simulink model "ADSBMonitor2020"  (R2020b)
settings: Solver=FixedStepDiscrete  StartTime=0.0  StopTime=inf  RelTol=1e-3
PreLoadFcn:
  | radioSampleRate = 2.4e6;
  | adsbParam = helperAdsbConfig(radioSampleRate);
  | load dataAdsbBusObjects
  | LaunchMap = 0;
  | LogData = 0;
  | BaudRate=9600;
InitFcn:
  | load dataAdsbBusObjects
  | helperAdsbCheckModelParams;
libraries: simrfV2util1 x3, simulink x2, instrumentlib x2, ADSBExampleLib x2, commsource2 x1, simrfV2systems x1, sdrrlib x1
CloseFcn:
  | hFig = findall(0, 'Type', 'figure', 'Tag', 'ADS-B Aircraft Tracking');
  | if ishghandle(hFig)
  | close(hFig);
  | end
  | clear hFig
settings Model: Creator=The MathWorks, Inc.  LastModifiedBy=Michael
settings DataIOCC: LimitDataPoints=on  SaveFormat=Array  SaveOutput=off  SaveTime=off  ReturnWorkspaceOutputs=off
settings OptimizationCC: BooleanDataType=off  DefaultParameterBehavior=Inlined  LocalBlockOutputs=off  LifeSpan=inf
settings DebuggingCC: AlgebraicLoopMsg=error  SingleTaskRateTransMsg=error  AllowSymbolicDim=off  SFUnexpectedBacktrackingDiag=warning  SFNoUnconditionalDefaultTransitionDiag=warning  SFExecutionAtInitializationDiag=none  ArithmeticOperatorsInVariantConditions=warning
settings ModelReferenceCC: PropagateSignalLabelsOutOfModel=off
settings SFSimCC: SimUseLocalCustomCode=off  CustomCodeUndefinedFunction=UseInterfaceOnly
settings RTWCC: RTWUseLocalCustomCode=off
settings CodeAppCC: StateflowObjectComments=on
settings GRTTargetCC: TargetLangStandard=C89/C90 (ANSI)
settings ConfigComp: CovScope=ReferencedModels  CovMetricSettings=dw  CovSaveCumulativeToWorkspaceVar=on  CovSaveSingleToWorkspaceVar=on  CovExternalEMLEnable=off  CovSFcnEnable=off

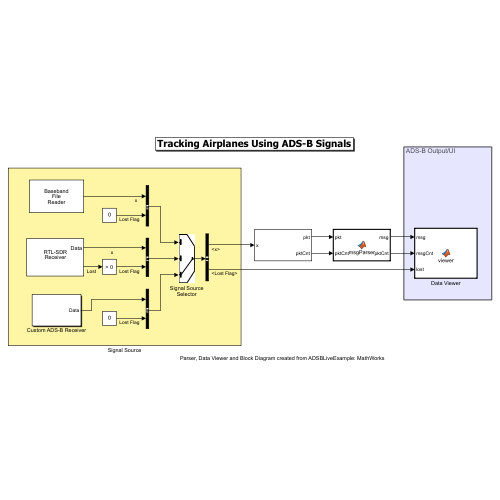
[thumbnail: Simulink's stored preview of the top-level diagram]
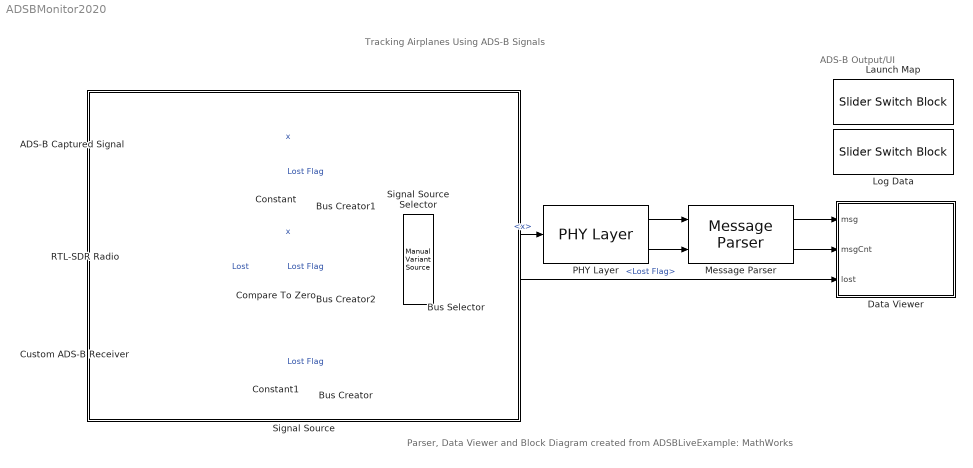
== system ADSBMonitor2020 ==
  note: ADS-B Output/UI
  note: Tracking Airplanes Using ADS-B Signals
  note: Parser, Data Viewer and Block Diagram created from ADSBLiveExample: MathWorks
  ADS-B Captured Signal : commsource2/Baseband File Reader  Filename=adsb_capture_01.bb  InheritSampleTimeFromFile=on  SampleTime=1  SamplesPerFrame=adsbParam.SamplesPerFrame  CyclicRepetition=on  FileEndOutputPort=off  SimulateUsing=Code generation
      settings: SourceProductBaseCode=CM
  Bus Creator : BusCreator  Inputs=2
  Bus Creator1 : BusCreator  Inputs=2
  Bus Creator2 : BusCreator  Inputs=2
  Bus Selector : BusSelector  OutputSignals=x,Lost Flag
  Compare To Zero : simulink/Logic and Bit Operations/Compare To Zero  relop=>  OutDataTypeStr=boolean
  Constant : Constant  Value=0
  Constant1 : Constant  Value=0
  Custom ADS-B Receiver : Subsystem
  Data Viewer : MATLAB Function  StopFcn=|  TreatAsAtomicUnit=on  mask(ADS-B viewer){logfilename=test.txt}
      | adsbGUI=findall(0,'type','figure','Tag','ADS-B Aircraft Tracking');
      | if ~isempty(adsbGUI)
      |   viewer=getappdata(adsbGUI,'ViewerHandle');
      |   stop(viewer);
      | end
      mask prompts: logfilename "Log data to file :"
  Launch Map : SliderSwitchBlock
      settings: Values={{'Off', 'On'}, [0 1]}
  Log Data : SliderSwitchBlock
      settings: Values={{'Off', 'On'}, [0 1]}
  Message Parser : ADSBExampleLib/Message Parser  SystemSampleTime=-1  VariantActivationTime=update diagram  Latency=0  AutoFrameSizeCalculation=off
  PHY Layer : ADSBExampleLib/PHY Layer  SystemSampleTime=-1  VariantActivationTime=update diagram  Latency=0  AutoFrameSizeCalculation=off
  RTL-SDR Radio : sdrrlib/RTL-SDR Receiver  IPAddress=0  CenterFrequencySource=Dialog  CenterFrequency=1090e6  GainSource=Dialog  Gain=60  ADCRate=adsbParam.FrontEndSampleRate  FrequencyCorrection=0  LostSamplesOutputPort=on  LatencyOutputPort=off  OutputDataType=single  FrameLength=adsbParam.SamplesPerFrame  EnableBurstMode=off  NumFramesInBurst=100  sobjType=sdrr.internal.SDRRTLReceiverSL  dataUDPPort=-1  ctrlUDPPort=-1  subDeviceList=nosubdev  sdrBlockType=SDRBlockTypeSLT.SDRRxBlock  requester=UNUSED_BY_SFCN  sdrExecutionMode=SDRExecutionModeSLT.ExecModeHW  BypassUserLogic=off  DecimatorSelect=DDC decimator  SourceSelect=RF data  SineAmplitude=16000  EnableInternalClock=off  BypassIQBalance=off  IFBandwidth=40e6  ADCRateSource=Dialog  IntermediateFrequency=0  DecimationFactorSource=Dialog  DecimationFactor=512  RFFrequencyIsTunable=logical(0)  SampleTime=(adsbParam.SamplesPerFrame)/(adsbParam.FrontEndSampleRate)  IFBandwidthSource=Dialog  SineFrequency=30000  BypassDCBlockingFilter=off  IntermediateFrequencySource=Dialog  IQBalanceCoefficients=64  SkipAllHardwareResetAndInitialization=off  EnableIQCalibrationTable=on  CacheIQCalibrationTable=off  EnableOffsetTuning=off  EnableRTLAGC=off  EnableTestMode=off  EnableTunerAGC=off  FrequencyCorrectionSource=Dialog  NumMLBuffers=128  NumUSBBuffers=16  RTLCrystalFrequency=28800000  TunerCrystalFrequency=28800000
      settings: SourceProductBaseCode=RTLSDR
  Signal Source : Subsystem
      mask Display: disp('')
  Signal Source Selector : simulink/Signal Routing/Manual Variant Source  NumChoices=3  LabelModeActiveChoice=V_3
  wires:
  Message Parser/1 -> Data Viewer/1(msg)
  Message Parser/2 -> Data Viewer/2(msgCnt)
  PHY Layer/1 -> Message Parser/1
  PHY Layer/2 -> Message Parser/2
  Bus Selector/2 -> Data Viewer/3(lost)  "<Lost Flag>"
  Bus Selector/1 -> PHY Layer/1  "<x>"
  RTL-SDR Radio/1 -> Bus Creator2/1  "x"
  ADS-B Captured Signal/1 -> Bus Creator1/1  "x"
  Bus Creator2/1 -> Signal Source Selector/2
  Signal Source Selector/1 -> Bus Selector/1
  Bus Creator/1 -> Signal Source Selector/3
  Bus Creator1/1 -> Signal Source Selector/1
  RTL-SDR Radio/2 -> Compare To Zero/1  "Lost"
  Compare To Zero/1 -> Bus Creator2/2  "Lost Flag"
  Constant/1 -> Bus Creator1/2  "Lost Flag"
  Constant1/1 -> Bus Creator/2  "Lost Flag"
  Custom ADS-B Receiver/1(Data) -> Bus Creator/1

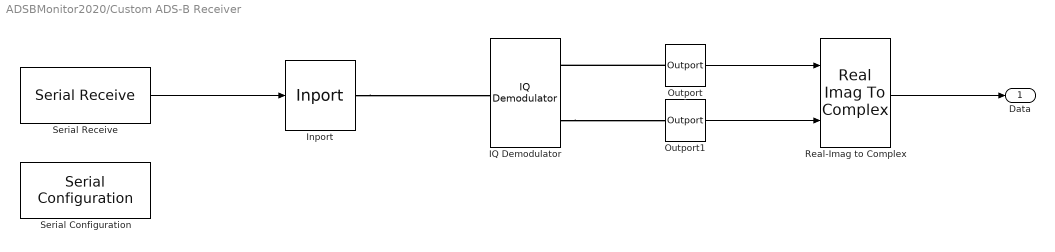
== system ADSBMonitor2020/Custom ADS-B Receiver ==
  IQ Demodulator : simrfV2systems/IQ Demodulator  classname=iqdemod  Source_linear_gain=Available power gain  linear_gain=0 dB  Poly_Coeffs=[0 1]  LOFreq=1090 MHz  Zin=50  Zout=50  AddIRFilter=off  AddCSFilters=off  InternalGrounding=on  ForceNextInit=off  Source_Poly=Even and odd order  IPType=Input  IP2=inf dBm  IP3=inf dBm  P1dB=inf dBm  Psat=inf dBm  Gcomp=inf dBm  NF=0  GainMismatch=0 dB  PhaseMismatch=0 deg  Isolation=inf dB  AddPhaseNoise=off  PhaseNoiseOffset=1  PhaseNoiseLevel=-Inf  AutoImpulseLengthPN=on  ImpulseLengthPN=1e-10  ImpulseLength_unitPN=s  DesignMethodIR=Ideal  ResponseTypeIR=Highpass  ImplementationIR=LC Tee  ImplementationIdealIR=Constant per carrier  ImplementationRationalIR=Transfer function  UseFilterOrderIR=on  FilterOrderIR=3  PassFreq_lpIR=1  PassFreq_lp_unitIR=GHz  PassFreq_hpIR=2  PassFreq_hp_unitIR=GHz  PassFreq_bpIR=[2 3]  PassFreq_bp_unitIR=GHz  PassFreq_bsIR=[1 4]  PassFreq_bs_unitIR=GHz  PassAttenIR=10*log10(2)  StopFreq_lpIR=2  StopFreq_lp_unitIR=GHz  StopFreq_hpIR=1  StopFreq_hp_unitIR=GHz  StopFreq_bpIR=[1.5 3.5]  StopFreq_bp_unitIR=GHz  StopFreq_bsIR=[2.1 2.9]  StopFreq_bs_unitIR=GHz  StopAttenIR=40  RsrcIR=50  RloadIR=50  AutoImpulseLengthIR=on  ImpulseLengthIR=1e-10  ImpulseLength_unitIR=s  DesignMethodCS=Ideal  ResponseTypeCS=Lowpass  ImplementationCS=LC Tee  ImplementationIdealCS=Constant per carrier  ImplementationRationalCS=Transfer function  UseFilterOrderCS=on  FilterOrderCS=3  PassFreq_lpCS=1  PassFreq_lp_unitCS=GHz  PassFreq_hpCS=2  PassFreq_hp_unitCS=GHz  PassFreq_bpCS=[2 3]  PassFreq_bp_unitCS=GHz  PassFreq_bsCS=[1 4]  PassFreq_bs_unitCS=GHz  PassAttenCS=10*log10(2)  StopFreq_lpCS=2  StopFreq_lp_unitCS=GHz  StopFreq_hpCS=1  StopFreq_hp_unitCS=GHz  StopFreq_bpCS=[1.5 3.5]  StopFreq_bp_unitCS=GHz  StopFreq_bsCS=[2.1 2.9]  StopFreq_bs_unitCS=GHz  StopAttenCS=40  RsrcCS=50  RloadCS=50  AutoImpulseLengthCS=on  ImpulseLengthCS=1e-10  ImpulseLength_unitCS=s
      settings: SourceProductBaseCode=RB
  Inport : simrfV2util1/Inport  SimulinkInputSignalType=Ideal voltage  CarrierFreq=1090 MHz  ZS=0  InternalGrounding=on
      settings: SourceProductBaseCode=RB
  Outport : simrfV2util1/Outport  SensorType=Ideal voltage  OutputFormat=Complex Baseband  CarrierFreq=0 Hz  ZL=Inf  InternalGrounding=on  StepSize=1e-6 s  AutoStep=on
      settings: SourceProductBaseCode=RB
  Outport1 : simrfV2util1/Outport  SensorType=Ideal voltage  OutputFormat=Complex Baseband  CarrierFreq=0 Hz  ZL=Inf  InternalGrounding=on  StepSize=1e-6 s  AutoStep=on
      settings: SourceProductBaseCode=RB
  Real-Imag to Complex : RealImagToComplex
  Serial Configuration : instrumentlib/Serial Configuration  Priority=-200000  ObjConstructor=serial('<Select a port...>');  ComPortMenu=<Please select a port...>  ComPort=<Please select a port...>  BaudRate=9600  DataBits=8  Parity=none  StopBits=1  ByteOrder=LittleEndian  FlowControl=none  Timeout=10
      settings: SourceProductBaseCode=OT,IC,MT
  Serial Receive : instrumentlib/Serial Receive  Priority=1  ObjConstructor=serial('<Select a port...>');  ComPortMenu=<Please select a port...>  ComPort=<Please select a port...>  DataType=uint16  DataSize=[1 1]  EnableBlockingMode=on  ActionDataUnavailable=Output last received value  CustomValue=0  SampleTime=0.01
      settings: SourceProductBaseCode=OT,IC,MT
  Data : Outport
  wires:
  Outport1/1 -> Real-Imag to Complex/2
  Real-Imag to Complex/1 -> Data/1
  Outport/1 -> Real-Imag to Complex/1
  Serial Receive/1 -> Inport/1
  connections:
  Outport/LConn1 -- IQ Demodulator/RConn1
  IQ Demodulator/RConn2 -- Outport1/LConn1
  Inport/RConn1 -- IQ Demodulator/LConn1

== system ADSBMonitor2020/Signal Source ==

== matlab function ADSBMonitor2020/Data Viewer ==
  data: msg input; msgCnt input; lost input; LaunchMap parameter; LogData parameter
function viewer(msg, msgCnt, lost, LaunchMap, LogData)
%#codegen

persistent resetGUI

if isempty(resetGUI)
  resetGUI = true;
end

block = 'ADSBMonitor/Data Viewer';

coder.extrinsic('helperAdsbViewerAdaptor');

coder.extrinsic('get_param','set_param');

Logfilename = get_param(block,'logfilename');

helperAdsbViewerAdaptor(msg, msgCnt, resetGUI, LaunchMap, LogData, Logfilename, lost);

resetGUI = false;
